simulink model "sampleModel1893_sub_sub"  (R2023a)
settings: Solver=VariableStepAuto  StartTime=0.0  StopTime=10.0  RelTol=1e-3
libraries: hdlsllib x6, simulink x4
settings Model: Creator=user1  LastModifiedBy=user1

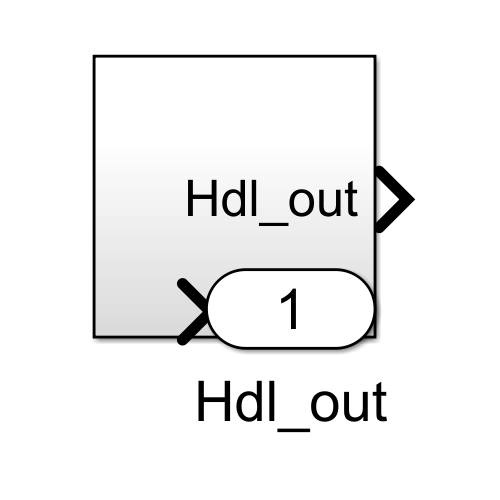
[thumbnail: Simulink's stored preview of the top-level diagram]
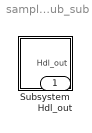
== system sampleModel1893_sub_sub ==
  Subsystem : Subsystem
  Hdl_out : Outport  OutDataTypeStr=uint8

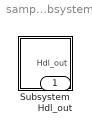
== system sampleModel1893_sub_sub/Subsystem ==
  Subsystem : Subsystem
  Hdl_out : Outport  OutDataTypeStr=uint8

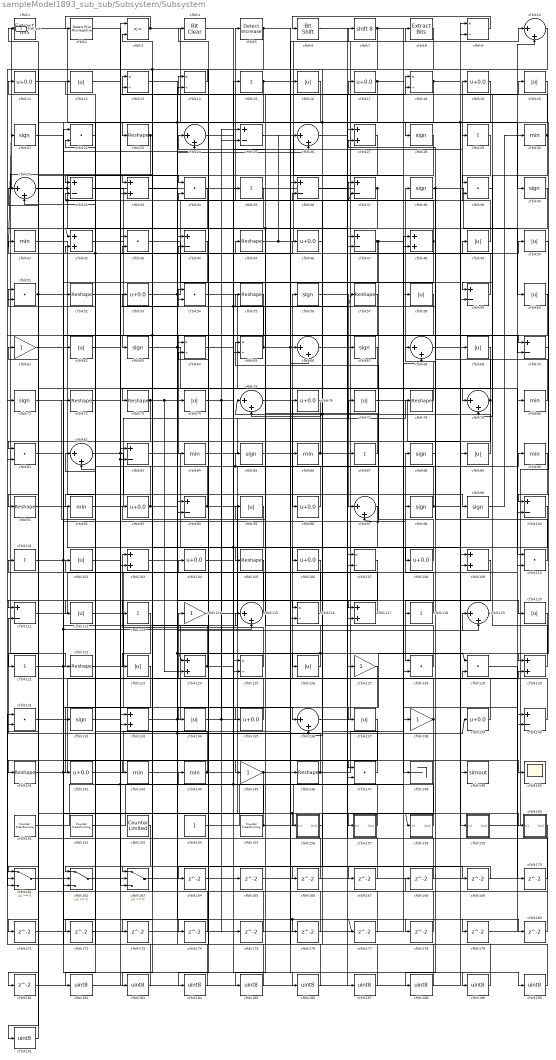
== system sampleModel1893_sub_sub/Subsystem/Subsystem ==
  cfblk1 : simulink/Logic and Bit Operations/Extract Bits  bitsToExtract=Upper half  numBits=8  bitIdxRange=[0 7]  outScalingMode=Preserve fixed-point scaling
      settings: LibrarySourceBlock=|
      | hdlsllib/Logic and Bit
      | Operations/Extract Bits
  cfblk{10,24,26,31,66,68,75,79,82,97,115,119,136} (13 alike) : Sum  Inputs=|++  OutDataTypeStr=uint8
  cfblk{25,32,36..37,44,47,59,70,83,94,100,111,140} (13 alike) : Sum  Inputs=+-  OutDataTypeStr=uint8
  cfblk{15,29,35,87,101,113,118,121} (8 alike) : Sum  Inputs=+  OutDataTypeStr=uint8
  cfblk{12,16,20,49..50,58,60,62,69,74,77,89,95,102,112,120,123,126,134,137} (20 alike) : Abs  OutDataTypeStr=uint8  SaturateOnIntegerOverflow=off
  cfblk{27,33,42,48,103,109,117,124,130,133} (10 alike) : Sum  OutDataTypeStr=uint8
  cfblk{11,17,19,46,53,76,93,96,104,106,108,135,139,142} (14 alike) : Bias  Bias=0.0  SaturateOnIntegerOverflow=off
  cfblk{23,45,52,55,57,72..73,78,91,105,122,141,146} (13 alike) : Reshape
  cfblk{9,13..14,18,64..65,107,116,125} (9 alike) : Product  Inputs=*/  OutDataTypeStr=uint8  RndMeth=Zero  SaturateOnIntegerOverflow=on
  cfblk{22,34,39,43,51,54,81,110,128..129,131,147} (12 alike) : DotProduct  OutDataTypeStr=uint8
  cfblk{61,114,127,138,145} (5 alike) : Gain  OutDataTypeStr=uint8
  cfblk{21,28,38,40,56,63,67,71,85,88,98..99,132} (13 alike) : Signum
  cfblk{30,41,80,84,86,90,92,143..144} (9 alike) : MinMax  OutDataTypeStr=uint8
  cfblk148 : Terminator
  cfblk149 : ToWorkspace  VariableName=simout  SaveFormat=Timeseries  SampleTime=-1
  cfblk150 : Scope
  cfblk151 : hdlsllib/Sources/Counter Free-Running  NumBits=16  tsamp=-1
  cfblk152 : hdlsllib/Sources/Counter Free-Running  NumBits=16  tsamp=-1
  cfblk153 : hdlsllib/Sources/Counter Limited  uplimit=7  tsamp=-1
  cfblk154 : Constant  OutDataTypeStr=uint8  SampleTime=-1
  cfblk155 : hdlsllib/Sources/Counter Free-Running  NumBits=16  tsamp=-1
  cfblk156 : Subsystem
      settings: LibrarySourceBlock=|
      | hdlsllib/Ports &
      | Subsystems/Subsystem
  cfblk157 : Subsystem
      settings: LibrarySourceBlock=|
      | hdlsllib/Ports &
      | Subsystems/Subsystem
  cfblk158 : Subsystem
      settings: LibrarySourceBlock=|
      | hdlsllib/Ports &
      | Subsystems/Subsystem
  cfblk159 : Subsystem
      settings: LibrarySourceBlock=|
      | hdlsllib/Ports &
      | Subsystems/Subsystem
  cfblk160 : Subsystem
      settings: LibrarySourceBlock=|
      | hdlsllib/Ports &
      | Subsystems/Subsystem
  cfblk161 : Switch  OutDataTypeStr=uint8  SaturateOnIntegerOverflow=off  InputSameDT=off
  cfblk162 : Switch  OutDataTypeStr=uint8  SaturateOnIntegerOverflow=off  InputSameDT=off
  cfblk163 : Switch  OutDataTypeStr=uint8  SaturateOnIntegerOverflow=off  InputSameDT=off
  cfblk{164..181} (18 alike) : Delay  SampleTime=1
  cfblk{182..191} (10 alike) : DataTypeConversion  OutDataTypeStr=uint8  SaturateOnIntegerOverflow=off  RndMeth=Floor
  cfblk2 : hdlsllib/Logic and Bit Operations/Detect Rise Nonnegative  vinit=0  OutDataTypeStr=uint8
  cfblk3 : RelationalOperator  Operator=<=  OutDataTypeStr=boolean  InputSameDT=off
  cfblk4 : simulink/Logic and Bit Operations/Bit Clear  iBit=0
      settings: LibrarySourceBlock=|
      | hdlsllib/Logic and Bit
      | Operations/Bit Clear
  cfblk5 : simulink/Logic and Bit Operations/Detect Increase  vinit=0.0  OutDataTypeStr=uint8
      settings: LibrarySourceBlock=|
      | hdlsllib/Logic and Bit
      | Operations/Detect
      | Increase
  cfblk6 : hdlsllib/Logic and Bit Operations/Bit Shift  mode=Shift Left Logical  N=0
  cfblk7 : ArithShift  BitShiftNumber=8
  cfblk8 : simulink/Logic and Bit Operations/Extract Bits  bitsToExtract=Upper half  numBits=8  bitIdxRange=[0 7]  outScalingMode=Preserve fixed-point scaling
      settings: LibrarySourceBlock=|
      | hdlsllib/Logic and Bit
      | Operations/Extract Bits
  Hdl_out : Outport  OutDataTypeStr=uint8
  wires:
  cfblk191/1 -> cfblk61/1
  cfblk69/1 -> cfblk191/1
  cfblk190/1 -> cfblk131/2
  cfblk61/1 -> cfblk190/1
  cfblk189/1 -> cfblk36/2
  cfblk188/1 -> cfblk36/1
  cfblk88/1 -> cfblk188/1
  cfblk187/1 -> cfblk131/1
  cfblk36/1 -> cfblk187/1
  cfblk186/1 -> cfblk44/1
  cfblk4/1 -> cfblk186/1
  cfblk185/1 -> cfblk4/1
  cfblk184/1 -> cfblk22/2
  cfblk127/1 -> cfblk184/1
  cfblk183/1 -> cfblk22/1
  cfblk182/1 -> cfblk89/1
  cfblk22/1 -> cfblk182/1
  cfblk181/1 -> cfblk133/2
  cfblk180/1 -> cfblk82/1
  cfblk85/1 -> cfblk180/1
  cfblk179/1 -> cfblk110/2
  cfblk178/1 -> cfblk31/1
  cfblk177/1 -> cfblk43/1
  cfblk176/1 -> cfblk3/2
  cfblk175/1 -> cfblk83/1
  cfblk174/1 -> cfblk163/2
  cfblk8/1 -> cfblk174/1
  cfblk173/1 -> cfblk68/2
  cfblk172/1 -> cfblk14/2
  cfblk171/1 -> cfblk48/1
  cfblk137/1 -> cfblk171/1
  cfblk170/1 -> cfblk47/1
  cfblk129/1 -> cfblk170/1
  cfblk169/1 -> cfblk163/1
  cfblk168/1 -> cfblk1/1
  cfblk160/1(Out1) -> cfblk168/1
  cfblk167/1 -> cfblk66/1
  cfblk64/1 -> cfblk167/1
  cfblk166/1 -> cfblk94/1
  cfblk165/1 -> cfblk9/1
  cfblk24/1 -> cfblk165/1
  cfblk164/1 -> cfblk140/1
  cfblk140/1 -> cfblk41/1
  cfblk72/1 -> cfblk3/1
  cfblk17/1 -> cfblk140/2, cfblk32/1
  cfblk62/1 -> cfblk39/2
  cfblk27/1 -> cfblk132/1
  cfblk120/1 -> cfblk137/1
  cfblk128/1 -> cfblk93/1
  cfblk12/1 -> cfblk74/1
  cfblk40/1 -> cfblk42/1, cfblk185/1
  cfblk130/1 -> cfblk18/2
  cfblk1/1 -> cfblk94/2, cfblk128/2
  cfblk47/1 -> cfblk97/2, cfblk79/1, cfblk136/2
  cfblk57/1 -> cfblk172/1, cfblk173/1
  cfblk80/1 -> cfblk27/2
  cfblk162/1 -> cfblk46/1
  cfblk63/1 -> cfblk148/1, cfblk179/1
  cfblk93/1 -> cfblk51/2, cfblk178/1
  cfblk98/1 -> cfblk149/1, cfblk31/2
  cfblk152/1 -> cfblk27/1
  cfblk103/1 -> cfblk118/1
  cfblk38/1 -> cfblk60/1, cfblk108/1
  cfblk55/1 -> cfblk64/1
  cfblk138/1 -> cfblk64/2, cfblk166/1
  cfblk21/1 -> cfblk65/2
  cfblk106/1 -> cfblk134/1
  cfblk30/1 -> cfblk14/1, cfblk79/2
  cfblk117/1 -> cfblk13/2
  cfblk123/1 -> cfblk142/1
  cfblk133/1 -> cfblk16/1, cfblk119/1
  cfblk107/1 -> cfblk161/3
  cfblk43/1 -> cfblk109/1
  cfblk100/1 -> cfblk113/1
  cfblk79/1 -> cfblk112/1, cfblk53/1
  cfblk108/1 -> cfblk65/1
  cfblk16/1 -> cfblk92/1
  cfblk95/1 -> cfblk125/2, cfblk164/1
  cfblk66/1 -> cfblk18/1
  cfblk116/1 -> cfblk95/1
  cfblk25/1 -> cfblk138/1
  cfblk92/1 -> cfblk78/1
  cfblk121/1 -> cfblk98/1, cfblk147/1
  cfblk89/1 -> cfblk13/1
  cfblk46/1 -> cfblk106/1
  cfblk145/1 -> cfblk37/1, cfblk181/1
  cfblk39/1 -> cfblk59/1
  cfblk54/1 -> cfblk110/1
  cfblk26/1 -> cfblk127/1
  cfblk143/1 -> cfblk139/1, cfblk119/2
  cfblk11/1 -> cfblk40/1, cfblk59/2
  cfblk20/1 -> cfblk126/1, cfblk91/1
  cfblk29/1 -> cfblk39/1
  cfblk58/1 -> cfblk161/2
  cfblk97/1 -> cfblk107/2
  cfblk84/1 -> cfblk77/1
  cfblk163/1 -> cfblk80/1
  cfblk18/1 -> cfblk9/2, cfblk162/3
  cfblk81/1 -> cfblk24/2
  cfblk73/1 -> cfblk120/1, cfblk124/2, cfblk161/1
  cfblk105/1 -> cfblk143/1
  cfblk151/1 -> cfblk15/1, cfblk58/1, cfblk33/2
  cfblk157/1(Out1) -> cfblk144/1
  cfblk115/1 -> cfblk101/1
  cfblk113/1 -> cfblk123/1
  cfblk154/1 -> cfblk86/1
  cfblk141/1 -> cfblk130/2, cfblk115/1
  cfblk42/1 -> cfblk84/1
  cfblk6/1 -> cfblk87/1
  cfblk59/1 -> cfblk21/1, cfblk12/1
  cfblk161/1 -> cfblk52/1
  cfblk156/1(Out1) -> cfblk76/1
  cfblk135/1 -> cfblk104/1
  cfblk7/1 -> cfblk33/1, cfblk121/1, cfblk70/2
  cfblk124/1 -> cfblk35/1, cfblk43/2
  cfblk112/1 -> cfblk136/1
  cfblk68/1 -> cfblk20/1
  cfblk142/1 -> cfblk66/2
  cfblk126/1 -> cfblk45/1, cfblk124/1
  cfblk101/1 -> cfblk176/1, cfblk177/1, cfblk62/1
  cfblk65/1 -> cfblk8/1, cfblk189/1, cfblk44/2
  cfblk104/1 -> cfblk57/1, cfblk29/1
  cfblk111/1 -> cfblk10/2
  cfblk50/1 -> cfblk130/1
  cfblk119/1 -> cfblk49/1
  cfblk90/1 -> cfblk100/2
  cfblk82/1 -> cfblk163/3, cfblk147/2
  cfblk70/1 -> cfblk100/1
  cfblk28/1 -> cfblk141/1
  cfblk155/1 -> cfblk107/1, cfblk42/2
  cfblk60/1 -> cfblk67/1
  cfblk56/1 -> cfblk97/1
  cfblk44/1 -> cfblk162/2
  cfblk131/1 -> cfblk114/1
  cfblk75/1 -> cfblk96/1
  cfblk3/1 -> cfblk146/1, cfblk2/1
  cfblk35/1 -> cfblk81/2
  cfblk19/1 -> cfblk73/1
  cfblk76/1 -> cfblk75/2
  cfblk91/1 -> cfblk117/2
  cfblk146/1 -> cfblk111/2, cfblk48/2
  cfblk153/1 -> cfblk162/1
  cfblk49/1 -> cfblk19/1
  cfblk122/1 -> cfblk69/1
  cfblk32/1 -> cfblk116/2
  cfblk109/1 -> cfblk128/1
  cfblk74/1 -> cfblk125/1, cfblk25/1, cfblk175/1
  cfblk144/1 -> cfblk102/1, cfblk129/2
  cfblk83/1 -> cfblk105/1
  cfblk71/1 -> cfblk158/1(In1), cfblk156/1(In1), cfblk115/2
  cfblk77/1 -> cfblk159/1(In1)
  cfblk87/1 -> cfblk24/1
  cfblk134/1 -> cfblk150/1, cfblk25/2
  cfblk96/1 -> cfblk51/1, cfblk85/1
  cfblk86/1 -> cfblk50/1, cfblk54/2
  cfblk52/1 -> cfblk70/1
  cfblk34/1 -> cfblk111/1
  cfblk51/1 -> cfblk81/1, cfblk135/1, cfblk11/1
  cfblk102/1 -> cfblk17/1
  cfblk33/1 -> cfblk160/1(In1)
  cfblk132/1 -> cfblk54/1
  cfblk10/1 -> cfblk116/1
  cfblk110/1 -> cfblk68/1
  cfblk67/1 -> cfblk145/1
  cfblk94/1 -> cfblk157/1(In1), cfblk32/2
  cfblk159/1(Out1) -> cfblk28/1
  cfblk139/1 -> cfblk56/1
  cfblk2/1 -> cfblk133/1
  cfblk5/1 -> cfblk117/1, cfblk23/1
  cfblk136/1 -> cfblk10/1
  cfblk158/1(Out1) -> cfblk72/1
  cfblk125/1 -> cfblk103/1
  cfblk14/1 -> cfblk71/1
  cfblk13/1 -> cfblk129/1, cfblk169/1
  cfblk118/1 -> cfblk88/1
  cfblk53/1 -> cfblk5/1, cfblk26/2
  cfblk114/1 -> cfblk90/1
  cfblk48/1 -> cfblk34/2, cfblk82/2
  cfblk15/1 -> cfblk122/1, cfblk109/2
  cfblk9/1 -> cfblk6/1
  cfblk23/1 -> cfblk103/2, cfblk83/2, cfblk183/1
  cfblk99/1 -> cfblk30/1
  cfblk37/1 -> cfblk63/1, Hdl_out/1
  cfblk147/1 -> cfblk75/1, cfblk55/1
  cfblk41/1 -> cfblk99/1
  cfblk45/1 -> cfblk7/1, cfblk26/1
  cfblk31/1 -> cfblk47/2, cfblk37/2, cfblk34/1
  cfblk78/1 -> cfblk38/1

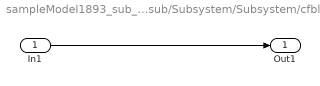
== system sampleModel1893_sub_sub/Subsystem/Subsystem/cfblk156 ==
  In1 : Inport
  Out1 : Outport
  wires:
  In1/1 -> Out1/1

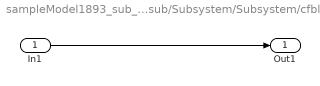
== system sampleModel1893_sub_sub/Subsystem/Subsystem/cfblk157 ==
  In1 : Inport
  Out1 : Outport
  wires:
  In1/1 -> Out1/1

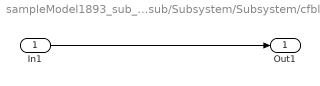
== system sampleModel1893_sub_sub/Subsystem/Subsystem/cfblk158 ==
  In1 : Inport
  Out1 : Outport
  wires:
  In1/1 -> Out1/1

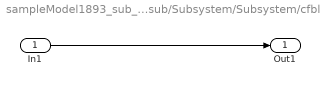
== system sampleModel1893_sub_sub/Subsystem/Subsystem/cfblk159 ==
  In1 : Inport
  Out1 : Outport
  wires:
  In1/1 -> Out1/1

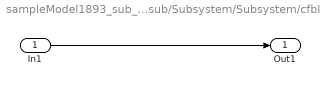
== system sampleModel1893_sub_sub/Subsystem/Subsystem/cfblk160 ==
  In1 : Inport
  Out1 : Outport
  wires:
  In1/1 -> Out1/1
